simulink model "gss10"  (Simulink 7.5)
settings: Solver=ode45  StartTime=0.0  StopTime=500  RelTol=1e-3
settings Model: Creator=Fer  LastModifiedBy=Fer
settings DebuggingCC: AlgebraicLoopMsg=none  SolverPrmCheckMsg=none  UnconnectedInputMsg=none  UnconnectedOutputMsg=none  UnconnectedLineMsg=none

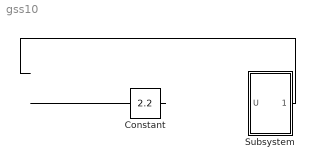
== system gss10 ==
  Constant : Constant  Value=2.2  OutDataType=fixdt(1, 16)  OutScaling=2^0
  Subsystem : Subsystem
  wires:
  ? -> Subsystem/1(U)
  Subsystem/1(Out1) -> ?
  Constant/1 -> ?

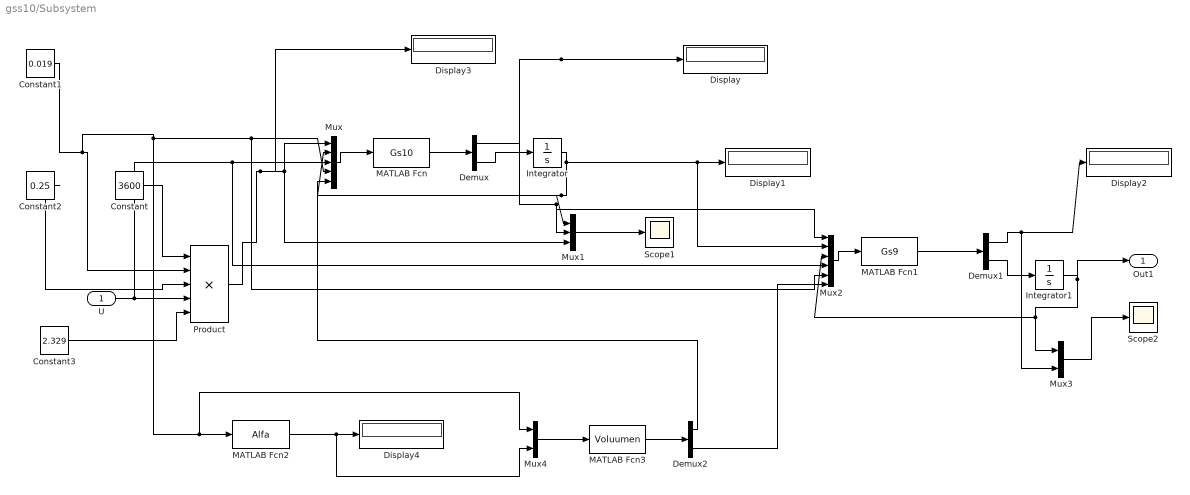
== system gss10/Subsystem ==
  U : Inport
  Constant : Constant  Value=3600  OutDataType=fixdt(1, 16)  OutScaling=2^0
  Constant1 : Constant  Value=0.019  OutDataType=fixdt(1, 16)  OutScaling=2^0
  Constant2 : Constant  Value=0.25  OutDataType=fixdt(1, 16)  OutScaling=2^0
  Constant3 : Constant  Value=2.329  OutDataType=fixdt(1, 16)  OutScaling=2^0
  Demux : Demux  Outputs=2
  Demux1 : Demux  Outputs=2
  Demux2 : Demux  Outputs=2
  Display{,1..4} (5 alike) : Display
  Integrator : Integrator  InitialCondition=1.6
  Integrator1 : Integrator  InitialCondition=1.6
  MATLAB Fcn : MATLABFcn  MATLABFcn=Gs10
  MATLAB Fcn1 : MATLABFcn  MATLABFcn=Gs9
  MATLAB Fcn2 : MATLABFcn  MATLABFcn=Alfa
  MATLAB Fcn3 : MATLABFcn  MATLABFcn=Voluumen
  Mux : Mux  Inputs=5
  Mux1 : Mux  Inputs=3
  Mux2 : Mux  Inputs=6
  Mux3 : Mux  Inputs=2
  Mux4 : Mux  Inputs=2
  Product : Product  Inputs=5  OutDataType=fixdt(1, 16)  OutScaling=2^0  RndMeth=Zero
  Scope1 : Scope
      settings: TimeRange=10  YMax=70
  Scope2 : Scope
      settings: TimeRange=100  YMin=0  YMax=25
  Out1 : Outport  OutDataType=fixdt(1, 16)  OutScaling=2^0
  wires:
  Integrator/1 -> Mux/2, Mux1/1, Display1/1, Mux2/2
  Mux/1 -> MATLAB Fcn/1
  MATLAB Fcn/1 -> Demux/1
  Demux/2 -> Integrator/1
  Demux/1 -> Display/1, Mux1/2, Mux2/1
  Mux1/1 -> Scope1/1
  Mux2/1 -> MATLAB Fcn1/1
  MATLAB Fcn1/1 -> Demux1/1
  Demux1/1 -> Display2/1, Mux3/2
  Demux1/2 -> Integrator1/1
  Integrator1/1 -> Mux3/1, Mux2/3, Out1/1
  Mux3/1 -> Scope2/1
  Product/1 -> Mux/1, Mux1/3, Display3/1
  Constant/1 -> Product/1
  Constant2/1 -> Product/3
  Constant3/1 -> Product/5
  MATLAB Fcn2/1 -> Display4/1, Mux4/2
  Mux4/1 -> MATLAB Fcn3/1
  MATLAB Fcn3/1 -> Demux2/1
  Demux2/1 -> Mux/5
  Demux2/2 -> Mux2/6
  Constant1/1 -> Product/2, Mux/4, Mux2/5, MATLAB Fcn2/1, Mux4/1
  U/1 -> Mux2/4, Mux/3, Product/4
